simulink model "Q2_melia"  (R2016a)
settings: Solver=VariableStepAuto  StartTime=0.0  StopTime=50e-3  RelTol=1e-3
libraries: powerlib x72, powerlib_meascontrol x17
settings Model: Creator=syf  LastModifiedBy=syf

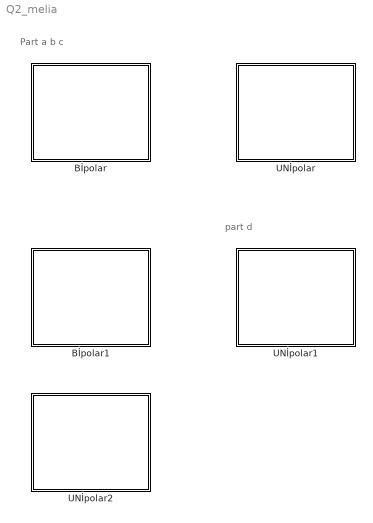
== system Q2_melia ==
  note: part d
  note: Part a b c
  Bİpolar : Subsystem
  Bİpolar1 : Subsystem
  UNİpolar : Subsystem
  UNİpolar1 : Subsystem
  UNİpolar2 : Subsystem

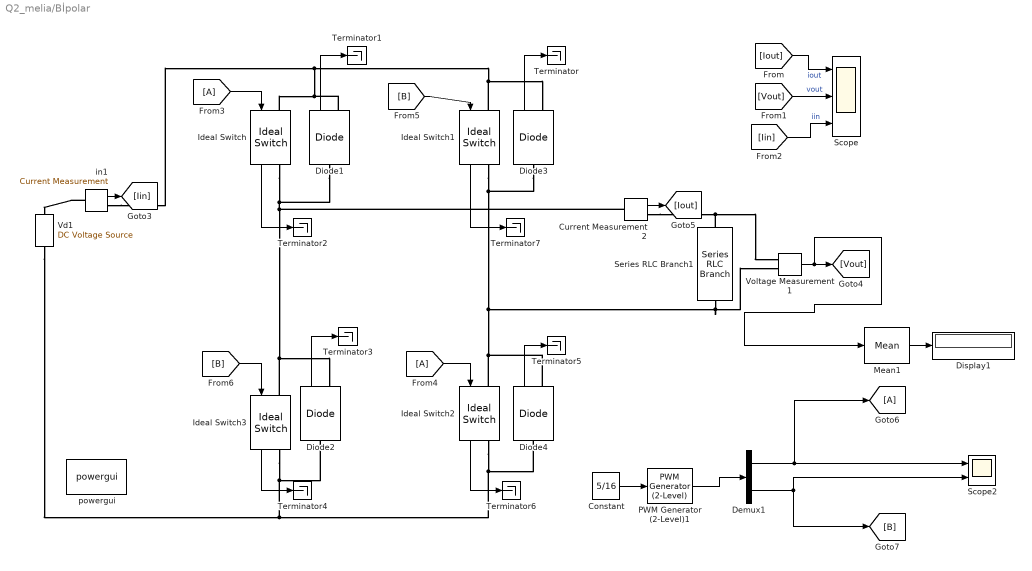
== system Q2_melia/Bİpolar ==
  Constant : Constant  Value=5/16
  Current Measurement2 : powerlib/Measurements/Current Measurement  PhasorSimulation=off  OutputType=Complex  PSBequivalent=0
  Demux1 : Demux  Outputs=2
  Diode{1..4} (4 alike) : powerlib/Power Electronics/Diode  Ron=0.001  Lon=0  Vf=0.8  IC=0  UseSnubber=off  Rs=500  Cs=250e-9  Measurements=on
  Display1 : Display
  Ideal Switch{,1..3} (4 alike) : powerlib/Power Electronics/Ideal Switch  Ron=0.001  Lon=0  IC=0  Rs=1e5  Cs=inf  Measurements=on
  Mean1 : powerlib_meascontrol/Measurements/Mean  Freq=20e3  Vinit=0  Ts=0
  PWM Generator (2-Level)1 : powerlib_meascontrol/Pulse & Signal Generators/PWM Generator (2-Level)  ModulatorType=Single-phase half-bridge (2 pulses)  ModulatorMode=Unsynchronized  Fc=20e3  Pc=0  nF=27  MinMax="[ -1  1 ]"  SamplingTechnique=Natural  ModulatingSignals=off  m=5/16  Freq=60  Phase=0  Ts=0  ShowCarrierOutport=off
  Scope : Scope  NumInputPorts=3
  Scope2 : Scope  NumInputPorts=2
  Series RLC Branch1 : powerlib/Elements/Series RLC Branch  LConnTagsString=__new0  RConnTagsString=__new0  BranchType=RL  Resistance=1.2  Inductance=3e-3  SetiL0=off  InitialCurrent=0  Capacitance=1e-6  Setx0=off  InitialVoltage=0  Measurements=None
  Terminator{,1..7} (8 alike) : Terminator
  Vd1 : powerlib/Electrical Sources/DC Voltage Source  Amplitude=48  Measurements=None
  Voltage Measurement1 : powerlib/Measurements/Voltage Measurement  PhasorSimulation=off  OutputType=Complex  PSBequivalent=0
  in1 : powerlib/Measurements/Current Measurement  PhasorSimulation=off  OutputType=Complex  PSBequivalent=0
  powergui : powerlib/powergui  Priority=1  SimulationMode=Continuous  SolverType=Tustin/Backward Euler (TBE)  SampleTime=50e-6  frequency=60  SPID=on  DisableSnubberDevices=off  DisableRonSwitches=off  DisableVfSwitches=on  SwTol=0  DisplayEquations=off  Interpol=off  ExternalGateDelay=off  methode=off  Ts=10  FunctionMessages=off  echomessages=off  HookPort=off  EnableUseOfTLC=off  x0status=blocks  frequencyindice=0  Pbase=100e6  ErrMax=1e-4  Iterations=50  UnitsV=kV  UnitsW=MW  buscounter=0  RestoreLinks=warning  ResistiveCurrentMeasurement=off  Frange=[0:2:500]  Ylog=off  Xlog=on  ShowGrid=off  save=off  variable=ZData  structure=0  ZoomFFT=off  StartTime=0.0  cycles=1  DisplayStyle=1  fundamental=60  FreqAxis=off  MaxFrequency=1000  frequencyindicesteady=1  RmsSteady=1  display=off
  wires:
  in1/1 -> [Iin]
  [B] -> Ideal Switch3/1
  Voltage Measurement1/1 -> Mean1/1, [Vout]
  Current Measurement2/1 -> [Iout]
  Mean1/1 -> Display1/1
  PWM Generator (2-Level)1/1 -> Demux1/1
  Constant/1 -> PWM Generator (2-Level)1/1
  [Vout] -> Scope/2  "vout"
  [Iout] -> Scope/1  "iout"
  [Iin] -> Scope/3  "iin"
  [B] -> Ideal Switch1/1
  [A] -> Ideal Switch/1
  [A] -> Ideal Switch2/1
  Diode4/1 -> Terminator5/1
  Diode2/1 -> Terminator3/1
  Diode3/1 -> Terminator/1
  Ideal Switch/1 -> Terminator2/1
  Diode1/1 -> Terminator1/1
  Ideal Switch3/1 -> Terminator4/1
  Ideal Switch2/1 -> Terminator6/1
  Demux1/2 -> [B], Scope2/2
  Demux1/1 -> [A], Scope2/1
  Ideal Switch1/1 -> Terminator7/1
  connections:
  in1/RConn1 -- Ideal Switch/LConn1 -- Diode1/RConn1 -- Diode3/RConn1 -- Ideal Switch1/LConn1
  in1/LConn1 -- Vd1/RConn1
  Series RLC Branch1/LConn1 -- Voltage Measurement1/LConn1 -- Current Measurement2/RConn1
  Ideal Switch1/RConn1 -- Diode3/LConn1 -- Series RLC Branch1/RConn1 -- Voltage Measurement1/LConn2 -- Diode4/RConn1 -- Ideal Switch2/LConn1
  Ideal Switch2/RConn1 -- Diode4/LConn1 -- Vd1/LConn1 -- Diode2/LConn1 -- Ideal Switch3/RConn1
  Ideal Switch/RConn1 -- Diode1/LConn1 -- Current Measurement2/LConn1 -- Diode2/RConn1 -- Ideal Switch3/LConn1

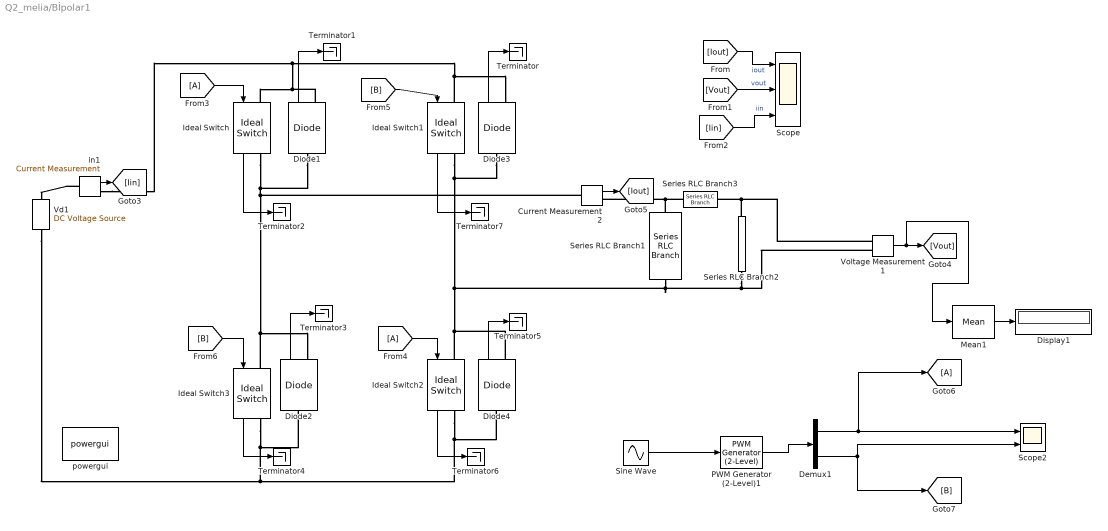
== system Q2_melia/Bİpolar1 ==
  Current Measurement2 : powerlib/Measurements/Current Measurement  PhasorSimulation=off  OutputType=Complex  PSBequivalent=0
  Demux1 : Demux  Outputs=2
  Diode{1..4} (4 alike) : powerlib/Power Electronics/Diode  Ron=0.001  Lon=0  Vf=0.8  IC=0  UseSnubber=off  Rs=500  Cs=250e-9  Measurements=on
  Display1 : Display
  Ideal Switch{,1..3} (4 alike) : powerlib/Power Electronics/Ideal Switch  Ron=0.001  Lon=0  IC=0  Rs=1e5  Cs=inf  Measurements=on
  Mean1 : powerlib_meascontrol/Measurements/Mean  Freq=20e3  Vinit=0  Ts=0
  PWM Generator (2-Level)1 : powerlib_meascontrol/Pulse & Signal Generators/PWM Generator (2-Level)  ModulatorType=Single-phase half-bridge (2 pulses)  ModulatorMode=Unsynchronized  Fc=20e3  Pc=0  nF=27  MinMax="[ -1  1 ]"  SamplingTechnique=Natural  ModulatingSignals=off  m=5/16  Freq=60  Phase=0  Ts=0  ShowCarrierOutport=off
  Scope : Scope  NumInputPorts=3
  Scope2 : Scope  NumInputPorts=2
  Series RLC Branch1 : powerlib/Elements/Series RLC Branch  LConnTagsString=__new0  RConnTagsString=__new0  BranchType=RL  Resistance=1.2  Inductance=3e-3  SetiL0=off  InitialCurrent=0  Capacitance=1e-6  Setx0=off  InitialVoltage=0  Measurements=None
  Series RLC Branch2 : powerlib/Elements/Series RLC Branch  LConnTagsString=__new0  RConnTagsString=__new0  BranchType=C  Resistance=1.2  Inductance=3e-3  SetiL0=off  InitialCurrent=0  Capacitance=47e-6  Setx0=off  InitialVoltage=0  Measurements=None
  Series RLC Branch3 : powerlib/Elements/Series RLC Branch  LConnTagsString=__new0  RConnTagsString=__new0  BranchType=L  Resistance=1.2  Inductance=33e-6  SetiL0=off  InitialCurrent=0  Capacitance=1e-6  Setx0=off  InitialVoltage=0  Measurements=None
  Sine Wave : Sin  Amplitude=36/48  Frequency=400  SampleTime=0
  Terminator{,1..7} (8 alike) : Terminator
  Vd1 : powerlib/Electrical Sources/DC Voltage Source  Amplitude=48  Measurements=None
  Voltage Measurement1 : powerlib/Measurements/Voltage Measurement  PhasorSimulation=off  OutputType=Complex  PSBequivalent=0
  in1 : powerlib/Measurements/Current Measurement  PhasorSimulation=off  OutputType=Complex  PSBequivalent=0
  powergui : powerlib/powergui  Priority=1  SimulationMode=Continuous  SolverType=Tustin/Backward Euler (TBE)  SampleTime=50e-6  frequency=60  SPID=on  DisableSnubberDevices=off  DisableRonSwitches=off  DisableVfSwitches=on  SwTol=0  DisplayEquations=off  Interpol=off  ExternalGateDelay=off  methode=off  Ts=10  FunctionMessages=off  echomessages=off  HookPort=off  EnableUseOfTLC=off  x0status=blocks  frequencyindice=0  Pbase=100e6  ErrMax=1e-4  Iterations=50  UnitsV=kV  UnitsW=MW  buscounter=0  RestoreLinks=warning  ResistiveCurrentMeasurement=off  Frange=[0:2:500]  Ylog=off  Xlog=on  ShowGrid=off  save=off  variable=ZData  structure=0  ZoomFFT=off  StartTime=0.0  cycles=1  DisplayStyle=1  fundamental=60  FreqAxis=off  MaxFrequency=1000  frequencyindicesteady=1  RmsSteady=1  display=off
  wires:
  Ideal Switch1/1 -> Terminator7/1
  Demux1/1 -> Scope2/1, [A]
  Demux1/2 -> Scope2/2, [B]
  Ideal Switch2/1 -> Terminator6/1
  Ideal Switch3/1 -> Terminator4/1
  Diode1/1 -> Terminator1/1
  Ideal Switch/1 -> Terminator2/1
  Diode3/1 -> Terminator/1
  Diode2/1 -> Terminator3/1
  Diode4/1 -> Terminator5/1
  [A] -> Ideal Switch2/1
  [A] -> Ideal Switch/1
  [B] -> Ideal Switch1/1
  [Iin] -> Scope/3  "iin"
  [Iout] -> Scope/1  "iout"
  [Vout] -> Scope/2  "vout"
  Sine Wave/1 -> PWM Generator (2-Level)1/1
  PWM Generator (2-Level)1/1 -> Demux1/1
  Mean1/1 -> Display1/1
  Current Measurement2/1 -> [Iout]
  Voltage Measurement1/1 -> [Vout], Mean1/1
  [B] -> Ideal Switch3/1
  in1/1 -> [Iin]
  connections:
  Ideal Switch3/LConn1 -- Diode2/RConn1 -- Current Measurement2/LConn1 -- Diode1/LConn1 -- Ideal Switch/RConn1
  Ideal Switch3/RConn1 -- Diode2/LConn1 -- Vd1/LConn1 -- Diode4/LConn1 -- Ideal Switch2/RConn1
  Ideal Switch2/LConn1 -- Diode4/RConn1 -- Series RLC Branch2/RConn1 -- Voltage Measurement1/LConn2 -- Series RLC Branch1/RConn1 -- Diode3/LConn1 -- Ideal Switch1/RConn1
  in1/LConn1 -- Vd1/RConn1
  Ideal Switch1/LConn1 -- Diode3/RConn1 -- Diode1/RConn1 -- Ideal Switch/LConn1 -- in1/RConn1
  Series RLC Branch1/LConn1 -- Series RLC Branch3/LConn1 -- Current Measurement2/RConn1
  Series RLC Branch2/LConn1 -- Series RLC Branch3/RConn1 -- Voltage Measurement1/LConn1

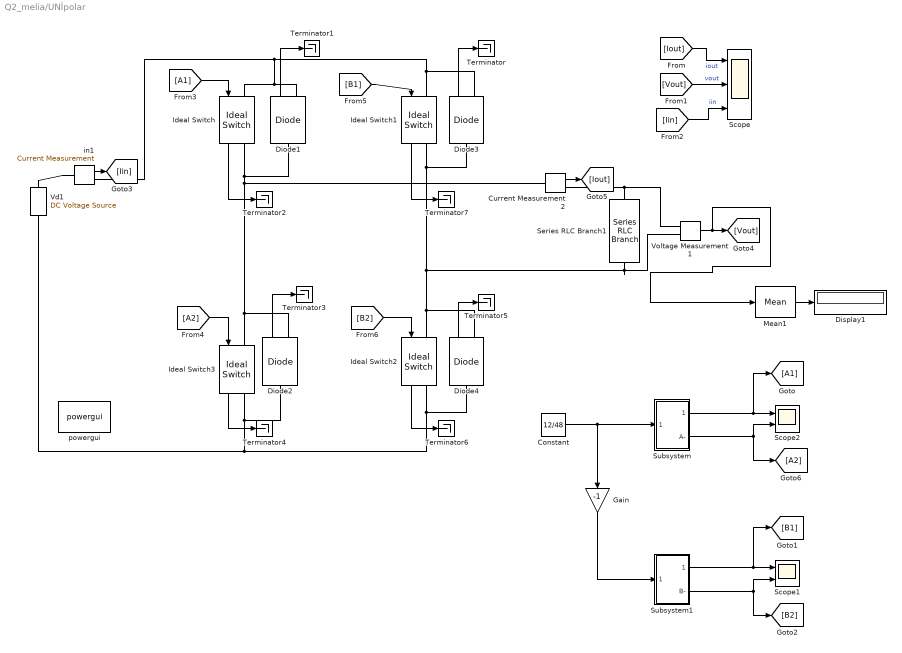
== system Q2_melia/UNİpolar ==
  Constant : Constant  Value=12/48
  Current Measurement2 : powerlib/Measurements/Current Measurement  PhasorSimulation=off  OutputType=Complex  PSBequivalent=0
  Diode{1..4} (4 alike) : powerlib/Power Electronics/Diode  Ron=0.001  Lon=0  Vf=0.8  IC=0  UseSnubber=off  Rs=500  Cs=250e-9  Measurements=on
  Display1 : Display
  Gain : Gain  Gain=-1
  Ideal Switch{,1..3} (4 alike) : powerlib/Power Electronics/Ideal Switch  Ron=0.001  Lon=0  IC=0  Rs=1e5  Cs=inf  Measurements=on
  Mean1 : powerlib_meascontrol/Measurements/Mean  Freq=20e3  Vinit=0  Ts=0
  Scope : Scope  NumInputPorts=3
  Scope1 : Scope  NumInputPorts=2
  Scope2 : Scope  NumInputPorts=2
  Series RLC Branch1 : powerlib/Elements/Series RLC Branch  LConnTagsString=__new0  RConnTagsString=__new0  BranchType=RL  Resistance=1.2  Inductance=3e-3  SetiL0=off  InitialCurrent=0  Capacitance=1e-6  Setx0=off  InitialVoltage=0  Measurements=None
  Subsystem : Subsystem
  Subsystem1 : Subsystem
  Terminator{,1..7} (8 alike) : Terminator
  Vd1 : powerlib/Electrical Sources/DC Voltage Source  Amplitude=48  Measurements=None
  Voltage Measurement1 : powerlib/Measurements/Voltage Measurement  PhasorSimulation=off  OutputType=Complex  PSBequivalent=0
  in1 : powerlib/Measurements/Current Measurement  PhasorSimulation=off  OutputType=Complex  PSBequivalent=0
  powergui : powerlib/powergui  Priority=1  SimulationMode=Continuous  SolverType=Tustin/Backward Euler (TBE)  SampleTime=50e-6  frequency=60  SPID=on  DisableSnubberDevices=off  DisableRonSwitches=off  DisableVfSwitches=on  SwTol=0  DisplayEquations=off  Interpol=off  ExternalGateDelay=off  methode=off  Ts=10  FunctionMessages=off  echomessages=off  HookPort=off  EnableUseOfTLC=off  x0status=blocks  frequencyindice=0  Pbase=100e6  ErrMax=1e-4  Iterations=50  UnitsV=kV  UnitsW=MW  buscounter=0  RestoreLinks=warning  ResistiveCurrentMeasurement=off  Frange=[0:2:500]  Ylog=off  Xlog=on  ShowGrid=off  save=off  variable=ZData  structure=0  ZoomFFT=off  StartTime=0.0  cycles=1  DisplayStyle=1  fundamental=60  FreqAxis=off  MaxFrequency=1000  frequencyindicesteady=1  RmsSteady=1  display=off
  wires:
  Ideal Switch1/1 -> Terminator7/1
  Ideal Switch2/1 -> Terminator6/1
  Ideal Switch3/1 -> Terminator4/1
  Diode1/1 -> Terminator1/1
  Ideal Switch/1 -> Terminator2/1
  Diode3/1 -> Terminator/1
  Diode2/1 -> Terminator3/1
  Diode4/1 -> Terminator5/1
  [B2] -> Ideal Switch2/1
  [A1] -> Ideal Switch/1
  [B1] -> Ideal Switch1/1
  [Iin] -> Scope/3  "iin"
  [Iout] -> Scope/1  "iout"
  [Vout] -> Scope/2  "vout"
  Mean1/1 -> Display1/1
  Current Measurement2/1 -> [Iout]
  Voltage Measurement1/1 -> [Vout], Mean1/1
  [A2] -> Ideal Switch3/1
  in1/1 -> [Iin]
  Subsystem/2(A-) -> [A2], Scope2/2
  Subsystem/1(A+) -> [A1], Scope2/1
  Constant/1 -> Gain/1, Subsystem/1(Duty)
  Subsystem1/2(B-) -> Scope1/2, [B2]
  Subsystem1/1(B+) -> Scope1/1, [B1]
  Gain/1 -> Subsystem1/1(Duty)
  connections:
  Ideal Switch3/LConn1 -- Diode2/RConn1 -- Current Measurement2/LConn1 -- Diode1/LConn1 -- Ideal Switch/RConn1
  Ideal Switch3/RConn1 -- Diode2/LConn1 -- Vd1/LConn1 -- Diode4/LConn1 -- Ideal Switch2/RConn1
  Ideal Switch2/LConn1 -- Diode4/RConn1 -- Voltage Measurement1/LConn2 -- Series RLC Branch1/RConn1 -- Diode3/LConn1 -- Ideal Switch1/RConn1
  Current Measurement2/RConn1 -- Voltage Measurement1/LConn1 -- Series RLC Branch1/LConn1
  in1/LConn1 -- Vd1/RConn1
  Ideal Switch1/LConn1 -- in1/RConn1 -- Diode1/RConn1 -- Ideal Switch/LConn1 -- Diode3/RConn1

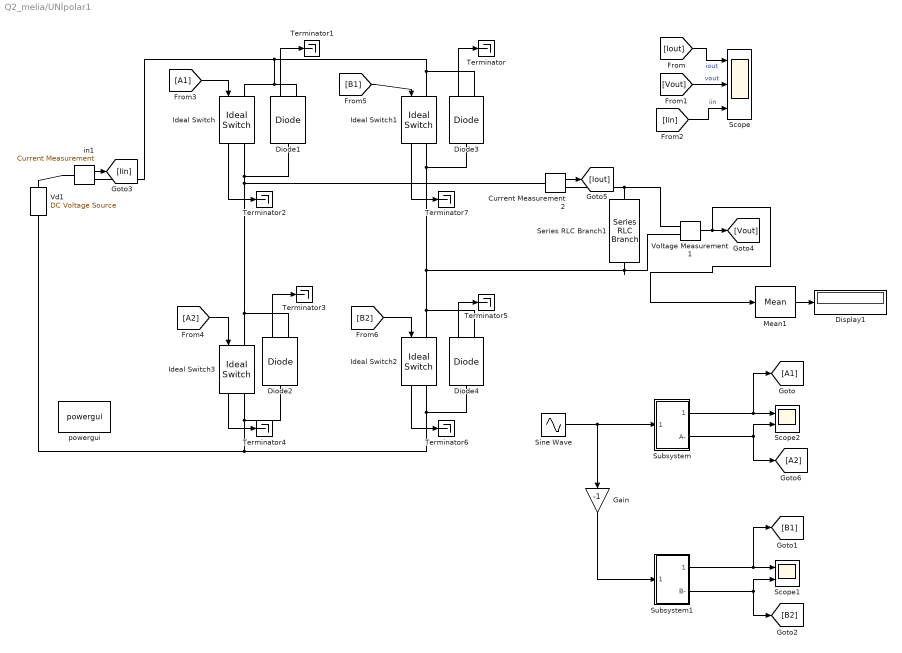
== system Q2_melia/UNİpolar1 ==
  Current Measurement2 : powerlib/Measurements/Current Measurement  PhasorSimulation=off  OutputType=Complex  PSBequivalent=0
  Diode{1..4} (4 alike) : powerlib/Power Electronics/Diode  Ron=0.001  Lon=0  Vf=0.8  IC=0  UseSnubber=off  Rs=500  Cs=250e-9  Measurements=on
  Display1 : Display
  Gain : Gain  Gain=-1
  Ideal Switch{,1..3} (4 alike) : powerlib/Power Electronics/Ideal Switch  Ron=0.001  Lon=0  IC=0  Rs=1e5  Cs=inf  Measurements=on
  Mean1 : powerlib_meascontrol/Measurements/Mean  Freq=20e3  Vinit=0  Ts=0
  Scope : Scope  NumInputPorts=3
  Scope1 : Scope  NumInputPorts=2
  Scope2 : Scope  NumInputPorts=2
  Series RLC Branch1 : powerlib/Elements/Series RLC Branch  LConnTagsString=__new0  RConnTagsString=__new0  BranchType=RL  Resistance=1.2  Inductance=3e-3  SetiL0=off  InitialCurrent=0  Capacitance=1e-6  Setx0=off  InitialVoltage=0  Measurements=None
  Sine Wave : Sin  Amplitude=36/48  SampleTime=0
  Subsystem : Subsystem
  Subsystem1 : Subsystem
  Terminator{,1..7} (8 alike) : Terminator
  Vd1 : powerlib/Electrical Sources/DC Voltage Source  Amplitude=48  Measurements=None
  Voltage Measurement1 : powerlib/Measurements/Voltage Measurement  PhasorSimulation=off  OutputType=Complex  PSBequivalent=0
  in1 : powerlib/Measurements/Current Measurement  PhasorSimulation=off  OutputType=Complex  PSBequivalent=0
  powergui : powerlib/powergui  Priority=1  SimulationMode=Continuous  SolverType=Tustin/Backward Euler (TBE)  SampleTime=50e-6  frequency=60  SPID=on  DisableSnubberDevices=off  DisableRonSwitches=off  DisableVfSwitches=on  SwTol=0  DisplayEquations=off  Interpol=off  ExternalGateDelay=off  methode=off  Ts=10  FunctionMessages=off  echomessages=off  HookPort=off  EnableUseOfTLC=off  x0status=blocks  frequencyindice=0  Pbase=100e6  ErrMax=1e-4  Iterations=50  UnitsV=kV  UnitsW=MW  buscounter=0  RestoreLinks=warning  ResistiveCurrentMeasurement=off  Frange=[0:2:500]  Ylog=off  Xlog=on  ShowGrid=off  save=off  variable=ZData  structure=0  ZoomFFT=off  StartTime=0.0  cycles=1  DisplayStyle=1  fundamental=60  FreqAxis=off  MaxFrequency=1000  frequencyindicesteady=1  RmsSteady=1  display=off
  wires:
  Gain/1 -> Subsystem1/1(Duty)
  Subsystem1/1(B+) -> [B1], Scope1/1
  Subsystem1/2(B-) -> [B2], Scope1/2
  Sine Wave/1 -> Subsystem/1(Duty), Gain/1
  Subsystem/1(A+) -> Scope2/1, [A1]
  Subsystem/2(A-) -> Scope2/2, [A2]
  in1/1 -> [Iin]
  [A2] -> Ideal Switch3/1
  Voltage Measurement1/1 -> Mean1/1, [Vout]
  Current Measurement2/1 -> [Iout]
  Mean1/1 -> Display1/1
  [Vout] -> Scope/2  "vout"
  [Iout] -> Scope/1  "iout"
  [Iin] -> Scope/3  "iin"
  [B1] -> Ideal Switch1/1
  [A1] -> Ideal Switch/1
  [B2] -> Ideal Switch2/1
  Diode4/1 -> Terminator5/1
  Diode2/1 -> Terminator3/1
  Diode3/1 -> Terminator/1
  Ideal Switch/1 -> Terminator2/1
  Diode1/1 -> Terminator1/1
  Ideal Switch3/1 -> Terminator4/1
  Ideal Switch2/1 -> Terminator6/1
  Ideal Switch1/1 -> Terminator7/1
  connections:
  Diode3/RConn1 -- Ideal Switch/LConn1 -- Diode1/RConn1 -- in1/RConn1 -- Ideal Switch1/LConn1
  in1/LConn1 -- Vd1/RConn1
  Series RLC Branch1/LConn1 -- Voltage Measurement1/LConn1 -- Current Measurement2/RConn1
  Ideal Switch1/RConn1 -- Diode3/LConn1 -- Series RLC Branch1/RConn1 -- Voltage Measurement1/LConn2 -- Diode4/RConn1 -- Ideal Switch2/LConn1
  Ideal Switch2/RConn1 -- Diode4/LConn1 -- Vd1/LConn1 -- Diode2/LConn1 -- Ideal Switch3/RConn1
  Ideal Switch/RConn1 -- Diode1/LConn1 -- Current Measurement2/LConn1 -- Diode2/RConn1 -- Ideal Switch3/LConn1

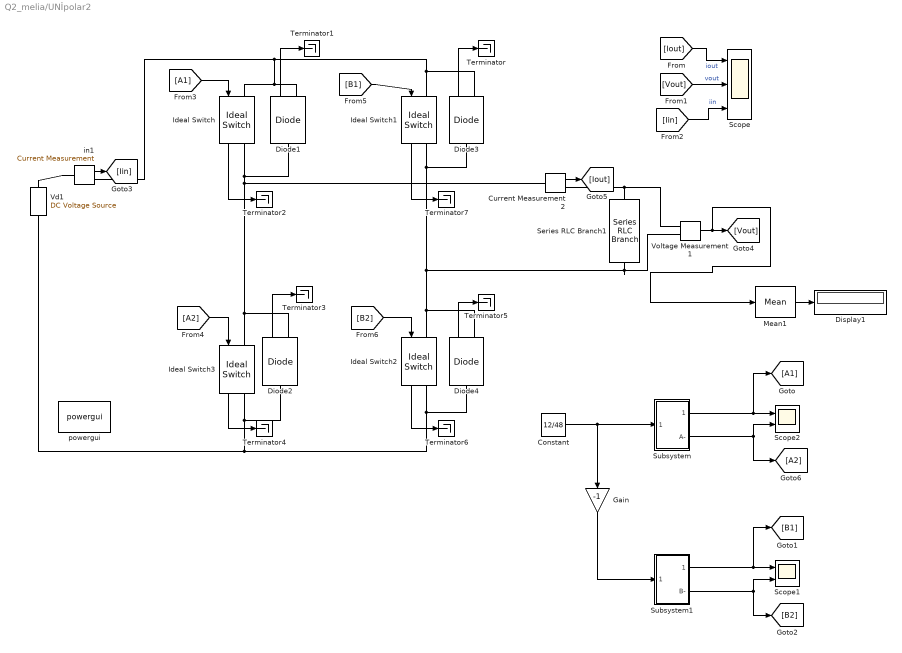
== system Q2_melia/UNİpolar2 ==
  Constant : Constant  Value=12/48
  Current Measurement2 : powerlib/Measurements/Current Measurement  PhasorSimulation=off  OutputType=Complex  PSBequivalent=0
  Diode{1..4} (4 alike) : powerlib/Power Electronics/Diode  Ron=0.001  Lon=0  Vf=0.8  IC=0  UseSnubber=off  Rs=500  Cs=250e-9  Measurements=on
  Display1 : Display
  Gain : Gain  Gain=-1
  Ideal Switch{,1..3} (4 alike) : powerlib/Power Electronics/Ideal Switch  Ron=0.001  Lon=0  IC=0  Rs=1e5  Cs=inf  Measurements=on
  Mean1 : powerlib_meascontrol/Measurements/Mean  Freq=20e3  Vinit=0  Ts=0
  Scope : Scope  NumInputPorts=3
  Scope1 : Scope  NumInputPorts=2
  Scope2 : Scope  NumInputPorts=2
  Series RLC Branch1 : powerlib/Elements/Series RLC Branch  LConnTagsString=__new0  RConnTagsString=__new0  BranchType=RL  Resistance=1.2  Inductance=3e-3  SetiL0=off  InitialCurrent=0  Capacitance=1e-6  Setx0=off  InitialVoltage=0  Measurements=None
  Subsystem : Subsystem
  Subsystem1 : Subsystem
  Terminator{,1..7} (8 alike) : Terminator
  Vd1 : powerlib/Electrical Sources/DC Voltage Source  Amplitude=48  Measurements=None
  Voltage Measurement1 : powerlib/Measurements/Voltage Measurement  PhasorSimulation=off  OutputType=Complex  PSBequivalent=0
  in1 : powerlib/Measurements/Current Measurement  PhasorSimulation=off  OutputType=Complex  PSBequivalent=0
  powergui : powerlib/powergui  Priority=1  SimulationMode=Continuous  SolverType=Tustin/Backward Euler (TBE)  SampleTime=50e-6  frequency=60  SPID=on  DisableSnubberDevices=off  DisableRonSwitches=off  DisableVfSwitches=on  SwTol=0  DisplayEquations=off  Interpol=off  ExternalGateDelay=off  methode=off  Ts=10  FunctionMessages=off  echomessages=off  HookPort=off  EnableUseOfTLC=off  x0status=blocks  frequencyindice=0  Pbase=100e6  ErrMax=1e-4  Iterations=50  UnitsV=kV  UnitsW=MW  buscounter=0  RestoreLinks=warning  ResistiveCurrentMeasurement=off  Frange=[0:2:500]  Ylog=off  Xlog=on  ShowGrid=off  save=off  variable=ZData  structure=0  ZoomFFT=off  StartTime=0.0  cycles=1  DisplayStyle=1  fundamental=60  FreqAxis=off  MaxFrequency=1000  frequencyindicesteady=1  RmsSteady=1  display=off
  wires:
  Gain/1 -> Subsystem1/1(Duty)
  Subsystem1/1(B+) -> [B1], Scope1/1
  Subsystem1/2(B-) -> [B2], Scope1/2
  Constant/1 -> Subsystem/1(Duty), Gain/1
  Subsystem/1(A+) -> Scope2/1, [A1]
  Subsystem/2(A-) -> Scope2/2, [A2]
  in1/1 -> [Iin]
  [A2] -> Ideal Switch3/1
  Voltage Measurement1/1 -> Mean1/1, [Vout]
  Current Measurement2/1 -> [Iout]
  Mean1/1 -> Display1/1
  [Vout] -> Scope/2  "vout"
  [Iout] -> Scope/1  "iout"
  [Iin] -> Scope/3  "iin"
  [B1] -> Ideal Switch1/1
  [A1] -> Ideal Switch/1
  [B2] -> Ideal Switch2/1
  Diode4/1 -> Terminator5/1
  Diode2/1 -> Terminator3/1
  Diode3/1 -> Terminator/1
  Ideal Switch/1 -> Terminator2/1
  Diode1/1 -> Terminator1/1
  Ideal Switch3/1 -> Terminator4/1
  Ideal Switch2/1 -> Terminator6/1
  Ideal Switch1/1 -> Terminator7/1
  connections:
  Diode3/RConn1 -- Ideal Switch/LConn1 -- Diode1/RConn1 -- in1/RConn1 -- Ideal Switch1/LConn1
  in1/LConn1 -- Vd1/RConn1
  Series RLC Branch1/LConn1 -- Voltage Measurement1/LConn1 -- Current Measurement2/RConn1
  Ideal Switch1/RConn1 -- Diode3/LConn1 -- Series RLC Branch1/RConn1 -- Voltage Measurement1/LConn2 -- Diode4/RConn1 -- Ideal Switch2/LConn1
  Ideal Switch2/RConn1 -- Diode4/LConn1 -- Vd1/LConn1 -- Diode2/LConn1 -- Ideal Switch3/RConn1
  Ideal Switch/RConn1 -- Diode1/LConn1 -- Current Measurement2/LConn1 -- Diode2/RConn1 -- Ideal Switch3/LConn1

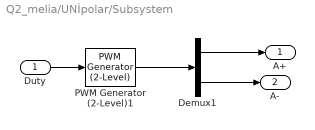
== system Q2_melia/UNİpolar/Subsystem ==
  Duty : Inport
  Demux1 : Demux  Outputs=2
  PWM Generator (2-Level)1 : powerlib_meascontrol/Pulse & Signal Generators/PWM Generator (2-Level)  ModulatorType=Single-phase half-bridge (2 pulses)  ModulatorMode=Unsynchronized  Fc=20e3  Pc=0  nF=27  MinMax="[ -1  1 ]"  SamplingTechnique=Natural  ModulatingSignals=off  m=5/16  Freq=60  Phase=0  Ts=0  ShowCarrierOutport=off
  A+ : Outport
  A- : Outport  Port=2
  wires:
  Demux1/2 -> A-/1
  Demux1/1 -> A+/1
  Duty/1 -> PWM Generator (2-Level)1/1
  PWM Generator (2-Level)1/1 -> Demux1/1

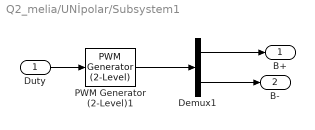
== system Q2_melia/UNİpolar/Subsystem1 ==
  Duty : Inport
  Demux1 : Demux  Outputs=2
  PWM Generator (2-Level)1 : powerlib_meascontrol/Pulse & Signal Generators/PWM Generator (2-Level)  ModulatorType=Single-phase half-bridge (2 pulses)  ModulatorMode=Unsynchronized  Fc=20e3  Pc=0  nF=27  MinMax="[ -1  1 ]"  SamplingTechnique=Natural  ModulatingSignals=off  m=5/16  Freq=60  Phase=0  Ts=0  ShowCarrierOutport=off
  B+ : Outport
  B- : Outport  Port=2
  wires:
  PWM Generator (2-Level)1/1 -> Demux1/1
  Duty/1 -> PWM Generator (2-Level)1/1
  Demux1/1 -> B+/1
  Demux1/2 -> B-/1

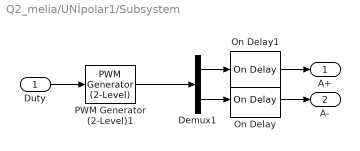
== system Q2_melia/UNİpolar1/Subsystem ==
  Duty : Inport
  Demux1 : Demux  Outputs=2
  On Delay : powerlib_meascontrol/Logic/On Delay  DelayType=On delay  delay=2e-6  ic=0  Ts=0
  On Delay1 : powerlib_meascontrol/Logic/On Delay  DelayType=On delay  delay=2e-6  ic=0  Ts=0
  PWM Generator (2-Level)1 : powerlib_meascontrol/Pulse & Signal Generators/PWM Generator (2-Level)  ModulatorType=Single-phase half-bridge (2 pulses)  ModulatorMode=Unsynchronized  Fc=20e3  Pc=0  nF=27  MinMax="[ -1  1 ]"  SamplingTechnique=Natural  ModulatingSignals=off  m=5/16  Freq=60  Phase=0  Ts=0  ShowCarrierOutport=off
  A+ : Outport
  A- : Outport  Port=2
  wires:
  PWM Generator (2-Level)1/1 -> Demux1/1
  Duty/1 -> PWM Generator (2-Level)1/1
  Demux1/1 -> On Delay1/1
  Demux1/2 -> On Delay/1
  On Delay/1 -> A-/1
  On Delay1/1 -> A+/1

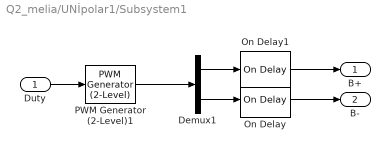
== system Q2_melia/UNİpolar1/Subsystem1 ==
  Duty : Inport
  Demux1 : Demux  Outputs=2
  On Delay : powerlib_meascontrol/Logic/On Delay  DelayType=On delay  delay=2e-6  ic=0  Ts=0
  On Delay1 : powerlib_meascontrol/Logic/On Delay  DelayType=On delay  delay=2e-6  ic=0  Ts=0
  PWM Generator (2-Level)1 : powerlib_meascontrol/Pulse & Signal Generators/PWM Generator (2-Level)  ModulatorType=Single-phase half-bridge (2 pulses)  ModulatorMode=Unsynchronized  Fc=20e3  Pc=0  nF=27  MinMax="[ -1  1 ]"  SamplingTechnique=Natural  ModulatingSignals=off  m=5/16  Freq=60  Phase=0  Ts=0  ShowCarrierOutport=off
  B+ : Outport
  B- : Outport  Port=2
  wires:
  Demux1/2 -> On Delay/1
  Demux1/1 -> On Delay1/1
  Duty/1 -> PWM Generator (2-Level)1/1
  PWM Generator (2-Level)1/1 -> Demux1/1
  On Delay/1 -> B-/1
  On Delay1/1 -> B+/1

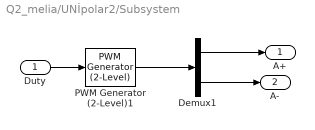
== system Q2_melia/UNİpolar2/Subsystem ==
  Duty : Inport
  Demux1 : Demux  Outputs=2
  PWM Generator (2-Level)1 : powerlib_meascontrol/Pulse & Signal Generators/PWM Generator (2-Level)  ModulatorType=Single-phase half-bridge (2 pulses)  ModulatorMode=Unsynchronized  Fc=20e3  Pc=0  nF=27  MinMax="[ -1  1 ]"  SamplingTechnique=Natural  ModulatingSignals=off  m=5/16  Freq=60  Phase=0  Ts=0  ShowCarrierOutport=off
  A+ : Outport
  A- : Outport  Port=2
  wires:
  PWM Generator (2-Level)1/1 -> Demux1/1
  Duty/1 -> PWM Generator (2-Level)1/1
  Demux1/1 -> A+/1
  Demux1/2 -> A-/1

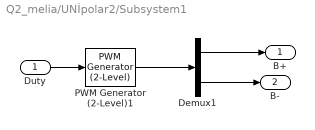
== system Q2_melia/UNİpolar2/Subsystem1 ==
  Duty : Inport
  Demux1 : Demux  Outputs=2
  PWM Generator (2-Level)1 : powerlib_meascontrol/Pulse & Signal Generators/PWM Generator (2-Level)  ModulatorType=Single-phase half-bridge (2 pulses)  ModulatorMode=Unsynchronized  Fc=20e3  Pc=0  nF=27  MinMax="[ -1  1 ]"  SamplingTechnique=Natural  ModulatingSignals=off  m=5/16  Freq=60  Phase=0  Ts=0  ShowCarrierOutport=off
  B+ : Outport
  B- : Outport  Port=2
  wires:
  Demux1/2 -> B-/1
  Demux1/1 -> B+/1
  Duty/1 -> PWM Generator (2-Level)1/1
  PWM Generator (2-Level)1/1 -> Demux1/1
